simulink model "untitled"  (Simulink 7.2)
settings: Solver=ode45  StartTime=0.0  StopTime=10.0  RelTol=1e-3
undefined symbols (not defined in the file or in its folder): b, bias, symmetric_aero_on
libraries: GTM_aerolib x3, aeroutilslib x2, engine_T2_lib x2, engine_JetCatP70_lib x2, aero_lib x1
settings Model: Creator=E183308  LastModifiedBy=E183308

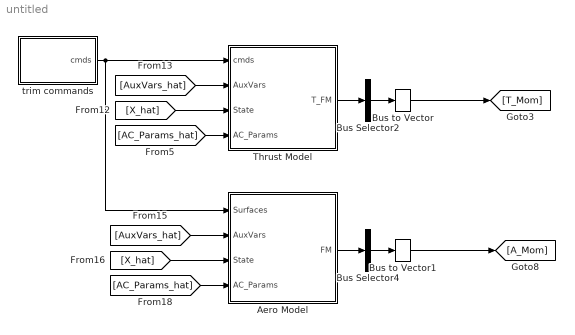
== system untitled ==
  Aero Model : Subsystem
  Bus Selector2 : BusSelector  OutputSignals=TLB,TMB,TNB  OutputAsBus=on
  Bus Selector4 : BusSelector  OutputSignals=LB,MB,NB  OutputAsBus=on
  Bus to Vector : BusToVector
  Bus to Vector1 : BusToVector
  Thrust Model : Subsystem
  trim commands : Subsystem
  wires:
  [X_hat] -> Thrust Model/3(State)
  [AuxVars_hat] -> Thrust Model/2(AuxVars)
  [AC_Params_hat] -> Thrust Model/4(AC_Params)
  trim commands/1(cmds) -> Thrust Model/1(cmds), Aero Model/1(Surfaces)
  [AuxVars_hat] -> Aero Model/2(AuxVars)
  [X_hat] -> Aero Model/3(State)
  [AC_Params_hat] -> Aero Model/4(AC_Params)
  Thrust Model/1(T_FM) -> Bus Selector2/1
  Bus Selector2/1 -> Bus to Vector/1
  Bus to Vector/1 -> [T_Mom]
  Bus Selector4/1 -> Bus to Vector1/1
  Bus to Vector1/1 -> [A_Mom]
  Aero Model/1(FM) -> Bus Selector4/1

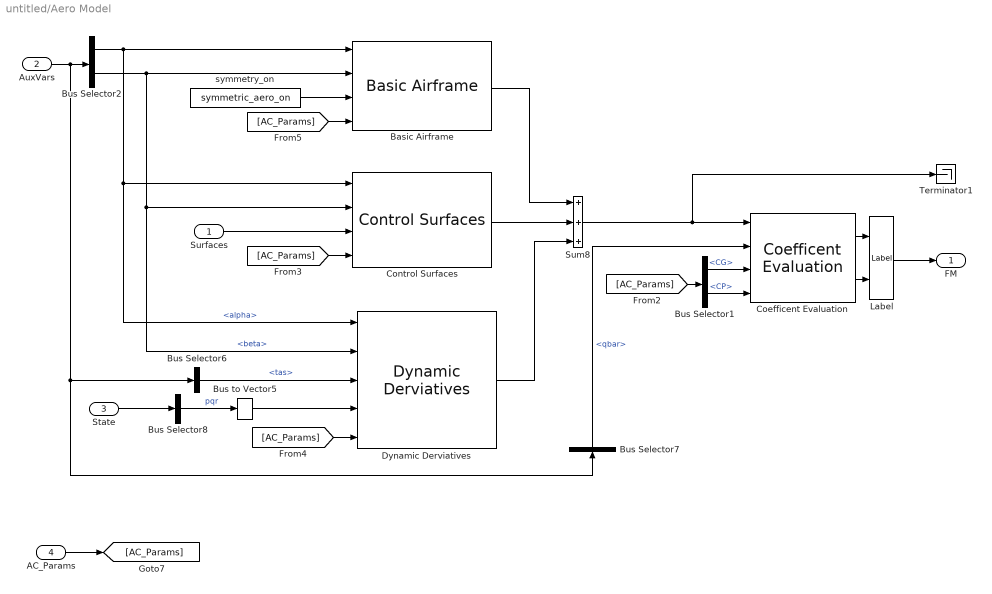
== system untitled/Aero Model ==
  Surfaces : Inport  OutDataType=sfix(16)  OutScaling=2^0
  AuxVars : Inport  Port=2  OutDataType=sfix(16)  OutScaling=2^0
  State : Inport  Port=3  OutDataType=sfix(16)  OutScaling=2^0
  AC_Params : Inport  Port=4  OutDataType=sfix(16)  OutScaling=2^0
  Basic Airframe : GTM_aerolib/Basic Airframe  SystemSampleTime=-1
  Bus Selector1 : BusSelector  OutputSignals=CG,CP
  Bus Selector2 : BusSelector  OutputSignals=alpha,beta
  Bus Selector6 : BusSelector  OutputSignals=tas
  Bus Selector7 : BusSelector  Orientation=up  OutputSignals=qbar
  Bus Selector8 : BusSelector  OutputSignals=pb,qb,rb  OutputAsBus=on
  Bus to Vector5 : BusToVector
  Coefficent Evaluation : aeroutilslib/Coefficent Evaluation  SystemSampleTime=-1  b=b  cbar=Cbar  Sref=S
  Control Surfaces : GTM_aerolib/Control Surfaces  SystemSampleTime=-1
  Dynamic Derviatives : GTM_aerolib/Dynamic Derviatives  SystemSampleTime=-1
  Label : aero_lib/GTM_T2/Label  SystemSampleTime=-1
  Sum8 : Sum  Inputs=+++  OutDataType=sfix(16)  OutScaling=2^0  SaturateOnIntegerOverflow=on  InputSameDT=on  OutDataTypeStr=Inherit: Same as first input
  Terminator1 : Terminator
  symmetry_on : Constant  Value=symmetric_aero_on  OutDataType=sfix(16)  OutScaling=2^0
  FM : Outport  OutDataType=sfix(16)  OutScaling=2^0
  wires:
  [AC_Params] -> Dynamic Derviatives/5
  Bus to Vector5/1 -> Dynamic Derviatives/4
  [AC_Params] -> Control Surfaces/4
  [AC_Params] -> Basic Airframe/4
  Bus Selector8/1 -> Bus to Vector5/1  "pqr"
  AC_Params/1 -> [AC_Params]
  Basic Airframe/1 -> Sum8/1
  Control Surfaces/1 -> Sum8/2
  Dynamic Derviatives/1 -> Sum8/3
  State/1 -> Bus Selector8/1
  Bus Selector2/2 -> Basic Airframe/2, Dynamic Derviatives/2, Control Surfaces/2  "<beta>"
  Bus Selector2/1 -> Basic Airframe/1, Dynamic Derviatives/1, Control Surfaces/1  "<alpha>"
  AuxVars/1 -> Bus Selector2/1, Bus Selector6/1, Bus Selector7/1
  Label/1 -> FM/1
  Bus Selector7/1 -> Coefficent Evaluation/2  "<qbar>"
  Sum8/1 -> Coefficent Evaluation/1, Terminator1/1
  Coefficent Evaluation/1 -> Label/1
  Coefficent Evaluation/2 -> Label/2
  Bus Selector1/1 -> Coefficent Evaluation/3  "<CG>"
  [AC_Params] -> Bus Selector1/1
  Bus Selector1/2 -> Coefficent Evaluation/4  "<CP>"
  symmetry_on/1 -> Basic Airframe/3
  Surfaces/1 -> Control Surfaces/3
  Bus Selector6/1 -> Dynamic Derviatives/3  "<tas>"

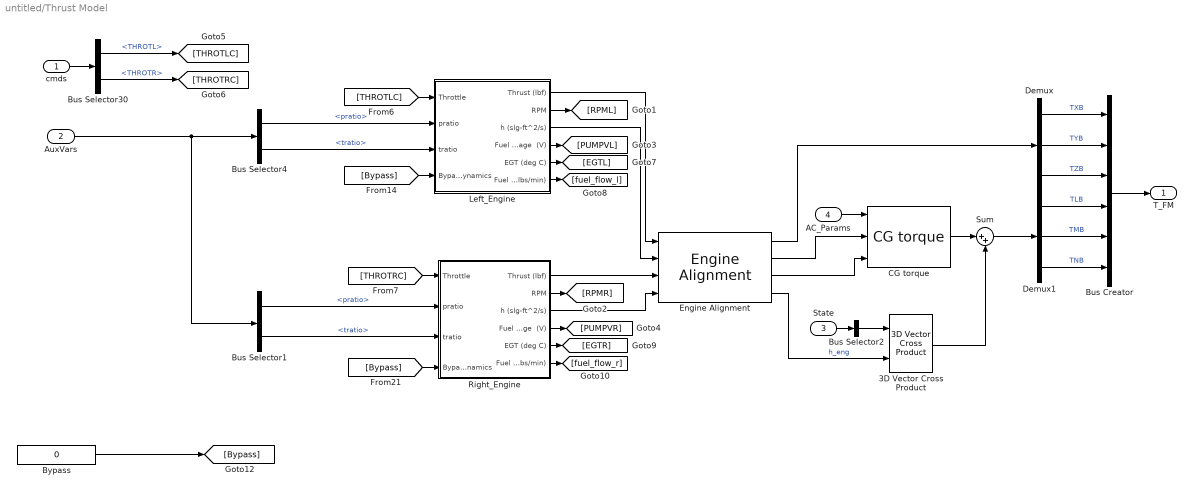
== system untitled/Thrust Model ==
  cmds : Inport  OutDataType=sfix(16)  OutScaling=2^0
  AuxVars : Inport  Port=2  OutDataType=sfix(16)  OutScaling=2^0
  State : Inport  Port=3  OutDataType=sfix(16)  OutScaling=2^0
  AC_Params : Inport  Port=4  OutDataType=sfix(16)  OutScaling=2^0
  3D Vector Cross Product : aeroutilslib/3D Vector Cross Product  SystemSampleTime=-1
  Bus Creator : BusCreator  Inputs=6
  Bus Selector1 : BusSelector  OutputSignals=pratio,tratio
  Bus Selector2 : BusSelector  OutputSignals=pb,qb,rb  OutputAsBus=on
  Bus Selector30 : BusSelector  OutputSignals=THROTL,THROTR
  Bus Selector4 : BusSelector  OutputSignals=pratio,tratio
  Bypass : Constant  Value=0  OutDataType=sfix(16)  OutScaling=2^0
  CG torque : engine_T2_lib/GTM_T2/CG torque  SystemSampleTime=-1
  Demux : Demux  Outputs=3
  Demux1 : Demux  Outputs=3
  Engine Alignment : engine_T2_lib/GTM_T2/Engine Alignment  SystemSampleTime=-1
  Left_Engine : Subsystem  BlockChoice=Jetcat P70
      settings: AttributesFormatString=%<BlockChoice>  TemplateBlock=enginelib/Engine Model  MemberBlocks=AMT-180,AMT-280,Blank,Jetcat P120SE,Jetcat P70
  Right_Engine : Subsystem  BlockChoice=Jetcat P70
      settings: AttributesFormatString=%<BlockChoice>  TemplateBlock=enginelib/Engine Model  MemberBlocks=AMT-180,AMT-280,Blank,Jetcat P120SE,Jetcat P70
  Sum : Sum  Inputs=|++  OutDataType=sfix(16)  OutScaling=2^0
  T_FM : Outport  PortDimensions=6  OutDataType=sfix(16)  OutScaling=2^0
  wires:
  Right_Engine/6(Fuel Flow (lbs/min)) -> [fuel_flow_r]
  Right_Engine/5(EGT (deg C)) -> [EGTR]
  Left_Engine/6(Fuel Flow (lbs/min)) -> [fuel_flow_l]
  Left_Engine/5(EGT (deg C)) -> [EGTL]
  cmds/1 -> Bus Selector30/1
  Demux/2 -> Bus Creator/2  "TYB"
  State/1 -> Bus Selector2/1
  Bus Selector2/1 -> 3D Vector Cross Product/1
  Demux/3 -> Bus Creator/3  "TZB"
  Left_Engine/2(RPM) -> [RPML]
  Left_Engine/4(Fuel Pump Voltage  (V)) -> [PUMPVL]
  Right_Engine/4(Fuel Pump Voltage  (V)) -> [PUMPVR]
  Right_Engine/2(RPM) -> [RPMR]
  Bus Selector1/1 -> Right_Engine/2(pratio)  "<pratio>"
  Bus Selector1/2 -> Right_Engine/3(tratio)  "<tratio>"
  AC_Params/1 -> CG torque/1
  Bus Creator/1 -> T_FM/1
  Bus Selector30/1 -> [THROTLC]  "<THROTL>"
  Bus Selector30/2 -> [THROTRC]  "<THROTR>"
  [THROTLC] -> Left_Engine/1(Throttle)
  [THROTRC] -> Right_Engine/1(Throttle)
  Bus Selector4/1 -> Left_Engine/2(pratio)  "<pratio>"
  Bus Selector4/2 -> Left_Engine/3(tratio)  "<tratio>"
  [Bypass] -> Left_Engine/4(BypassDynamics)
  [Bypass] -> Right_Engine/4(BypassDynamics)
  Bypass/1 -> [Bypass]
  Left_Engine/1(Thrust (lbf)) -> Engine Alignment/1
  Right_Engine/1(Thrust (lbf)) -> Engine Alignment/3
  Demux/1 -> Bus Creator/1  "TXB"
  Left_Engine/3(h (slg-ft^2/s)) -> Engine Alignment/2
  Right_Engine/3(h (slg-ft^2/s)) -> Engine Alignment/4
  Engine Alignment/4 -> 3D Vector Cross Product/2  "h_eng"
  Engine Alignment/1 -> Demux/1
  Engine Alignment/2 -> CG torque/2
  Engine Alignment/3 -> CG torque/3
  CG torque/1 -> Sum/1
  3D Vector Cross Product/1 -> Sum/2
  Sum/1 -> Demux1/1
  Demux1/1 -> Bus Creator/4  "TLB"
  Demux1/2 -> Bus Creator/5  "TMB"
  Demux1/3 -> Bus Creator/6  "TNB"
  AuxVars/1 -> Bus Selector1/1, Bus Selector4/1

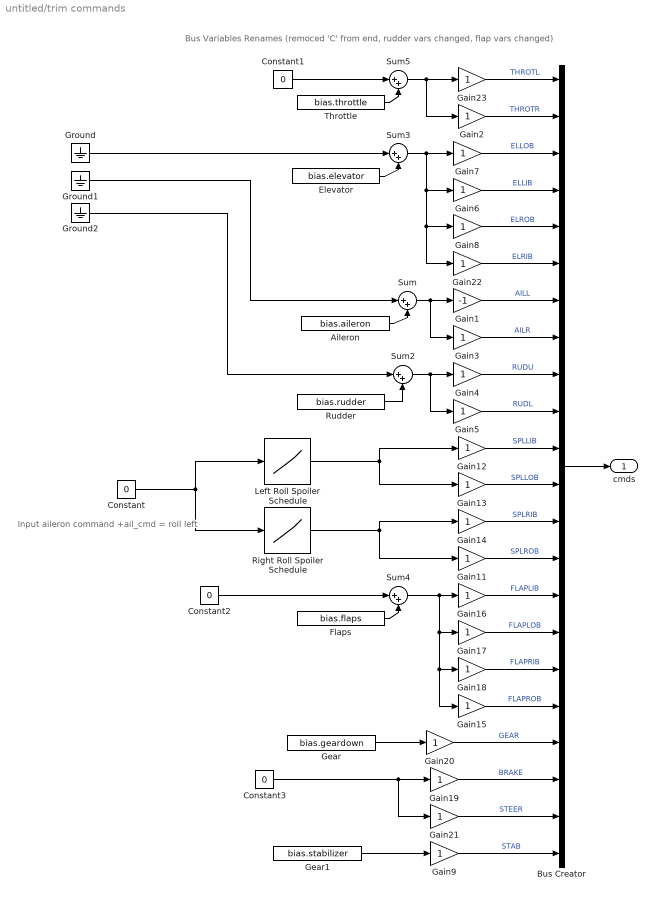
== system untitled/trim commands ==
  note: Input aileron command
      | +ail_cmd = roll left
  note: Bus Variables Renames (remoced 'C' from end, rudder vars changed, flap vars changed)
  Aileron : Constant  Value=bias.aileron  OutDataType=sfix(16)  OutScaling=2^0
  Bus Creator : BusCreator  Inputs=22
  Constant{,1..3} (4 alike) : Constant  Value=0  OutDataType=sfix(16)  OutScaling=2^0
  Elevator : Constant  Value=bias.elevator  OutDataType=sfix(16)  OutScaling=2^0
  Flaps : Constant  Value=bias.flaps  OutDataType=sfix(16)  OutScaling=2^0
  Gain1 : Gain  Gain=-1  ParameterDataType=sfix(16)  ParameterScaling=2^0  OutDataType=sfix(16)  OutScaling=2^0  SaturateOnIntegerOverflow=on  OutDataTypeStr=Inherit: Same as input  ParamDataTypeStr=Inherit: Same as input
  Gain{2..9,11..23} (21 alike) : Gain  ParameterDataType=sfix(16)  ParameterScaling=2^0  OutDataType=sfix(16)  OutScaling=2^0  SaturateOnIntegerOverflow=on  OutDataTypeStr=Inherit: Same as input  ParamDataTypeStr=Inherit: Same as input
  Gear : Constant  Value=bias.geardown  OutDataType=sfix(16)  OutScaling=2^0
  Gear1 : Constant  Value=bias.stabilizer  OutDataType=sfix(16)  OutScaling=2^0
  Ground : Ground
  Ground1 : Ground
  Ground2 : Ground
  Left Roll Spoiler Schedule : Lookup  InputValues="[-20\t-11.76\t-2.36\t0\t2.36\t11.76\t20\t]"  Table=[0 0 0 0 0 9 45]  LookUpMeth=Interpolation-Use End Values  OutDataType=sfix(16)  OutScaling=2^0
  Right Roll Spoiler Schedule : Lookup  InputValues="[-20\t-11.76\t-2.36\t0\t2.36\t11.76\t20\t]"  Table=[45 9 0 0 0 0 0]  LookUpMeth=Interpolation-Use End Values  OutDataType=sfix(16)  OutScaling=2^0
  Rudder : Constant  Value=bias.rudder  OutDataType=sfix(16)  OutScaling=2^0
  Sum{,2..5} (5 alike) : Sum  Inputs=|++  OutDataType=sfix(16)  OutScaling=2^0
  Throttle : Constant  Value=bias.throttle  OutDataType=sfix(16)  OutScaling=2^0
  cmds : Outport  OutDataType=sfix(16)  OutScaling=2^0
  wires:
  Right Roll Spoiler Schedule/1 -> Gain11/1, Gain14/1
  Left Roll Spoiler Schedule/1 -> Gain13/1, Gain12/1
  Gain12/1 -> Bus Creator/11  "SPLLIB"
  Gain13/1 -> Bus Creator/12  "SPLLOB"
  Gain14/1 -> Bus Creator/13  "SPLRIB"
  Gain11/1 -> Bus Creator/14  "SPLROB"
  Gain16/1 -> Bus Creator/15  "FLAPLIB"
  Gain17/1 -> Bus Creator/16  "FLAPLOB"
  Gain18/1 -> Bus Creator/17  "FLAPRIB"
  Gain15/1 -> Bus Creator/18  "FLAPROB"
  Gain23/1 -> Bus Creator/1  "THROTL"
  Gain2/1 -> Bus Creator/2  "THROTR"
  Gain6/1 -> Bus Creator/4  "ELLIB"
  Gain7/1 -> Bus Creator/3  "ELLOB"
  Gain8/1 -> Bus Creator/5  "ELROB"
  Gain22/1 -> Bus Creator/6  "ELRIB"
  Gain1/1 -> Bus Creator/7  "AILL"
  Gain3/1 -> Bus Creator/8  "AILR"
  Gain4/1 -> Bus Creator/9  "RUDU"
  Gain5/1 -> Bus Creator/10  "RUDL"
  Sum3/1 -> Gain7/1, Gain6/1, Gain8/1, Gain22/1
  Aileron/1 -> Sum/2
  Elevator/1 -> Sum3/2
  Sum/1 -> Gain1/1, Gain3/1
  Sum2/1 -> Gain4/1, Gain5/1
  Rudder/1 -> Sum2/2
  Flaps/1 -> Sum4/2
  Constant2/1 -> Sum4/1
  Sum4/1 -> Gain16/1, Gain17/1, Gain18/1, Gain15/1
  Ground1/1 -> Sum/1
  Ground2/1 -> Sum2/1
  Gain19/1 -> Bus Creator/20  "BRAKE"
  Gear/1 -> Gain20/1
  Constant3/1 -> Gain19/1, Gain21/1
  Bus Creator/1 -> cmds/1
  Gain20/1 -> Bus Creator/19  "GEAR"
  Gain21/1 -> Bus Creator/21  "STEER"
  Ground/1 -> Sum3/1
  Constant/1 -> Right Roll Spoiler Schedule/1, Left Roll Spoiler Schedule/1
  Throttle/1 -> Sum5/2
  Constant1/1 -> Sum5/1
  Sum5/1 -> Gain2/1, Gain23/1
  Gear1/1 -> Gain9/1
  Gain9/1 -> Bus Creator/22  "STAB"

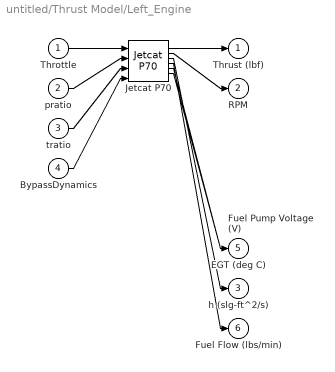
== system untitled/Thrust Model/Left_Engine ==
  Throttle : Inport  OutDataType=sfix(16)  OutScaling=2^0
  pratio : Inport  Port=2  OutDataType=sfix(16)  OutScaling=2^0
  tratio : Inport  Port=3  OutDataType=sfix(16)  OutScaling=2^0
  BypassDynamics : Inport  Port=4  OutDataType=sfix(16)  OutScaling=2^0
  Jetcat P70 : engine_JetCatP70_lib/Jetcat P70  SystemSampleTime=-1
  Thrust (lbf) : Outport  OutDataType=sfix(16)  OutScaling=2^0
  RPM : Outport  Port=2  OutDataType=sfix(16)  OutScaling=2^0
  h (slg-ft^2/s) : Outport  Port=3  OutDataType=sfix(16)  OutScaling=2^0
  Fuel Pump Voltage  (V) : Outport  Port=4  OutDataType=sfix(16)  OutScaling=2^0
  EGT (deg C) : Outport  Port=5  OutDataType=sfix(16)  OutScaling=2^0
  Fuel Flow (lbs/min) : Outport  Port=6  OutDataType=sfix(16)  OutScaling=2^0
  wires:
  Throttle/1 -> Jetcat P70/1
  pratio/1 -> Jetcat P70/2
  tratio/1 -> Jetcat P70/3
  BypassDynamics/1 -> Jetcat P70/4
  Jetcat P70/1 -> Thrust (lbf)/1
  Jetcat P70/2 -> RPM/1
  Jetcat P70/3 -> h (slg-ft^2/s)/1
  Jetcat P70/4 -> Fuel Flow (lbs/min)/1
  Jetcat P70/5 -> Fuel Pump Voltage  (V)/1
  Jetcat P70/6 -> EGT (deg C)/1

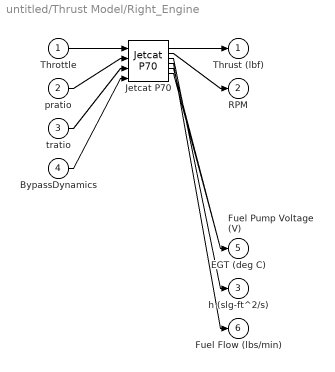
== system untitled/Thrust Model/Right_Engine ==
  Throttle : Inport  OutDataType=sfix(16)  OutScaling=2^0
  pratio : Inport  Port=2  OutDataType=sfix(16)  OutScaling=2^0
  tratio : Inport  Port=3  OutDataType=sfix(16)  OutScaling=2^0
  BypassDynamics : Inport  Port=4  OutDataType=sfix(16)  OutScaling=2^0
  Jetcat P70 : engine_JetCatP70_lib/Jetcat P70  SystemSampleTime=-1
  Thrust (lbf) : Outport  OutDataType=sfix(16)  OutScaling=2^0
  RPM : Outport  Port=2  OutDataType=sfix(16)  OutScaling=2^0
  h (slg-ft^2/s) : Outport  Port=3  OutDataType=sfix(16)  OutScaling=2^0
  Fuel Pump Voltage  (V) : Outport  Port=4  OutDataType=sfix(16)  OutScaling=2^0
  EGT (deg C) : Outport  Port=5  OutDataType=sfix(16)  OutScaling=2^0
  Fuel Flow (lbs/min) : Outport  Port=6  OutDataType=sfix(16)  OutScaling=2^0
  wires:
  Throttle/1 -> Jetcat P70/1
  pratio/1 -> Jetcat P70/2
  tratio/1 -> Jetcat P70/3
  BypassDynamics/1 -> Jetcat P70/4
  Jetcat P70/1 -> Thrust (lbf)/1
  Jetcat P70/2 -> RPM/1
  Jetcat P70/3 -> h (slg-ft^2/s)/1
  Jetcat P70/4 -> Fuel Flow (lbs/min)/1
  Jetcat P70/5 -> Fuel Pump Voltage  (V)/1
  Jetcat P70/6 -> EGT (deg C)/1
